simulink model "example_CollectorUnglazed_2node"  (R2018b)
settings: Solver=ode45  StartTime=0.0  StopTime=24*3600  RelTol=1e-5  AbsTol=1e-5  EnableMultiTasking=on
undefined symbols (not defined in the file): path_carnot
libraries: carnot x5
settings Model: Creator=drhf  LastModifiedBy=drhf
settings SolverCC: AutoScaleAbsTol=off
settings DataIOCC: LimitDataPoints=on  SaveFormat=Array
settings OptimizationCC: ExpressionDepthLimit=2147483647  LifeSpan=inf
settings DebuggingCC: UnderspecifiedInitializationDetection=Classic  MergeDetectMultiDrivingBlocksExec=none  SolverPrmCheckMsg=warning  StateNameClashWarn=warning  SFUnexpectedBacktrackingDiag=warning  SFNoUnconditionalDefaultTransitionDiag=warning  SFExecutionAtInitializationDiag=none
settings HardwareCC: ProdBitPerPointer=32  ProdBitPerSizeT=32  ProdBitPerPtrDiffT=32  ProdLargestAtomicFloat=None  ProdIntDivRoundTo=Undefined  ProdEndianess=Unspecified  ProdWordSize=32  ProdHWDeviceType=32-bit Generic
settings ModelReferenceCC: PropagateSignalLabelsOutOfModel=off
settings SFSimCC: SimUseLocalCustomCode=off
settings RTWCC: RTWUseLocalCustomCode=off
settings CodeAppCC: StateflowObjectComments=on
settings GRTTargetCC: TargetLangStandard=C89/C90 (ANSI)  GeneratePreprocessorConditionals=Disable all  CombineOutputUpdateFcns=off  GRTInterface=on
settings ConfigComp: CovMetricSettings=dw  CovHtmlReporting=on  CovSaveCumulativeToWorkspaceVar=on  CovSaveSingleToWorkspaceVar=on  CovExternalEMLEnable=off

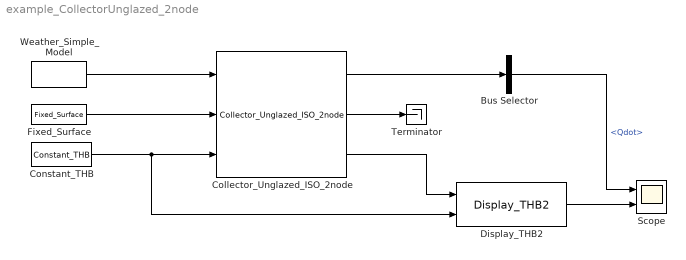
== system example_CollectorUnglazed_2node ==
  Bus Selector : BusSelector  OutputSignals=Qdot
  Collector_Unglazed_ISO_2node : carnot/Source/Solar_Thermal/Collector_Unglazed_ISO_2node  tini=20  Ncollector=1  PathName=fullfile(path_carnot('libsl'), 'Source', 'Solar_Thermal', 'Collector_Unglazed_ISO_2node', 'parameter_set')  FileName='Viessmann_SLK_ISO9806.mat'  userPath=off  userParam=off  acol=2.544  len=2.1  eta0=0.702  bu=0.066  b1=32.64  b2=3.59  c_abs=50*3900  dplin=5504.4  dpqua=6222.096
      settings: SourceProductName=Carnot
  Constant_THB : carnot/Source/Simple/Constant_THB  t=10  mdot=100/3600  p=1e5  mID=No Pressure Drop  fluid=Water  mix=0  mix2=0  mix3=0  dia=0.02  hgt=0
      settings: SourceProductName=Carnot
  Display_THB2 : carnot/Outputs/Display_THB2  t=on  m=off  p=off  id=off  mix=off  d=off
      settings: SourceProductName=Carnot
  Fixed_Surface : carnot/Weather/Fixed_Surface  colangle=30  colazi=0  colrot=0
      settings: SourceProductName=Carnot
  Scope : Scope  NumInputPorts=2
  Terminator : Terminator
  Weather_Simple_Model : carnot/Weather/Weather_Simple_Model  Ibn=900  Idg=100  tamb=5  deltaTsky=-6  rh=50  precip="10e-3/24/3600           % 10 mm in 24 h"  cloud=0.125  p=1013e2  vw=1  wdir=270  lat=60  colangle=0  colazi=0  colrot=0
      settings: SourceProductName=Carnot
  wires:
  Weather_Simple_Model/1 -> Collector_Unglazed_ISO_2node/1
  Fixed_Surface/1 -> Collector_Unglazed_ISO_2node/2
  Constant_THB/1 -> Collector_Unglazed_ISO_2node/3, Display_THB2/2
  Collector_Unglazed_ISO_2node/3 -> Display_THB2/1
  Display_THB2/1 -> Scope/2
  Collector_Unglazed_ISO_2node/1 -> Bus Selector/1
  Bus Selector/1 -> Scope/1  "<Qdot>"
  Collector_Unglazed_ISO_2node/2 -> Terminator/1
